simulink model "vel_estimator"  (R2024b)
settings: Solver=VariableStepAuto  StartTime=0.0  StopTime=10.0  RelTol=1e-3
settings Model: Creator=lukec  LastModifiedBy=lukec

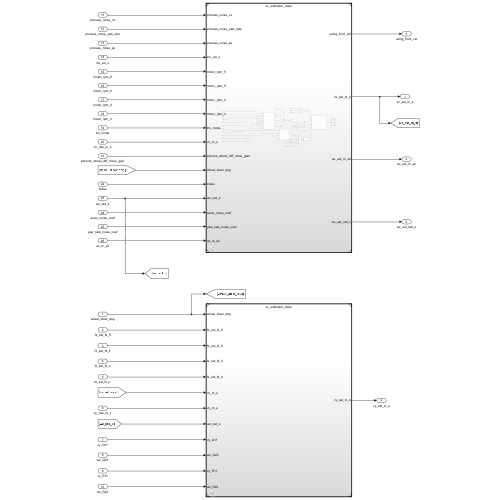
[thumbnail: Simulink's stored preview of the top-level diagram]
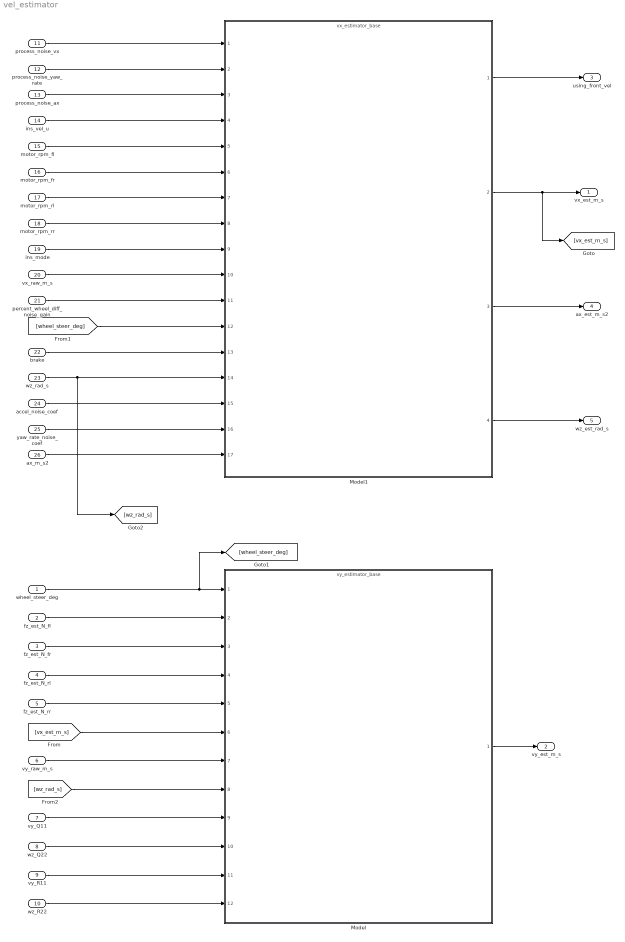
== system vel_estimator ==
  wheel_steer_deg : Inport
  fz_est_N_fl : Inport  Port=2
  fz_est_N_fr : Inport  Port=3
  fz_est_N_rl : Inport  Port=4
  fz_est_N_rr : Inport  Port=5
  vy_raw_m_s : Inport  Port=6
  vy_Q11 : Inport  Port=7
  wz_Q22 : Inport  Port=8
  vy_R11 : Inport  Port=9
  wz_R22 : Inport  Port=10
  process_noise_vx : Inport  Port=11
  process_noise_yaw_rate : Inport  Port=12
  process_noise_ax : Inport  Port=13
  ins_vel_u : Inport  Port=14
  motor_rpm_fl : Inport  Port=15
  motor_rpm_fr : Inport  Port=16
  motor_rpm_rl : Inport  Port=17
  motor_rpm_rr : Inport  Port=18
  ins_mode : Inport  Port=19
  vx_raw_m_s : Inport  Port=20
  percent_wheel_diff_noise_gain : Inport  Port=21
  brake : Inport  Port=22
  wz_rad_s : Inport  Port=23
  accel_noise_coef : Inport  Port=24
  yaw_rate_noise_coef : Inport  Port=25
  ax_m_s2 : Inport  Port=26
  Model : ModelReference  ModelNameDialog=vy_estimator_base.slx  SimulationMode=Normal  ModelReferenceVersion=1.5
  Model1 : ModelReference  ModelNameDialog=vx_estimator_base.slx  SimulationMode=Normal  ModelReferenceVersion=1.42
  vx_est_m_s : Outport
  vy_est_m_s : Outport  Port=2
  using_front_vel : Outport  Port=3
  ax_est_m_s2 : Outport  Port=4
  wz_est_rad_s : Outport  Port=5
  wires:
  fz_est_N_fl/1 -> Model/2
  fz_est_N_fr/1 -> Model/3
  fz_est_N_rl/1 -> Model/4
  fz_est_N_rr/1 -> Model/5
  [wz_rad_s] -> Model/8
  [vx_est_m_s] -> Model/6
  vy_raw_m_s/1 -> Model/7
  vy_R11/1 -> Model/11
  vy_Q11/1 -> Model/9
  wz_Q22/1 -> Model/10
  wz_R22/1 -> Model/12
  Model/1 -> vy_est_m_s/1
  process_noise_vx/1 -> Model1/1
  process_noise_yaw_rate/1 -> Model1/2
  process_noise_ax/1 -> Model1/3
  ins_vel_u/1 -> Model1/4
  motor_rpm_fl/1 -> Model1/5
  motor_rpm_fr/1 -> Model1/6
  motor_rpm_rl/1 -> Model1/7
  motor_rpm_rr/1 -> Model1/8
  ins_mode/1 -> Model1/9
  vx_raw_m_s/1 -> Model1/10
  percent_wheel_diff_noise_gain/1 -> Model1/11
  wheel_steer_deg/1 -> [wheel_steer_deg], Model/1
  [wheel_steer_deg] -> Model1/12
  brake/1 -> Model1/13
  wz_rad_s/1 -> [wz_rad_s], Model1/14
  accel_noise_coef/1 -> Model1/15
  yaw_rate_noise_coef/1 -> Model1/16
  ax_m_s2/1 -> Model1/17
  Model1/2 -> vx_est_m_s/1, [vx_est_m_s]
  Model1/1 -> using_front_vel/1
  Model1/3 -> ax_est_m_s2/1
  Model1/4 -> wz_est_rad_s/1
